simulink model "ModelResonant"  (R2020b)
settings: Solver=ode45  StartTime=0.0  StopTime=5  RelTol=1e-3
settings Model: Creator=umberto  LastModifiedBy=umberto

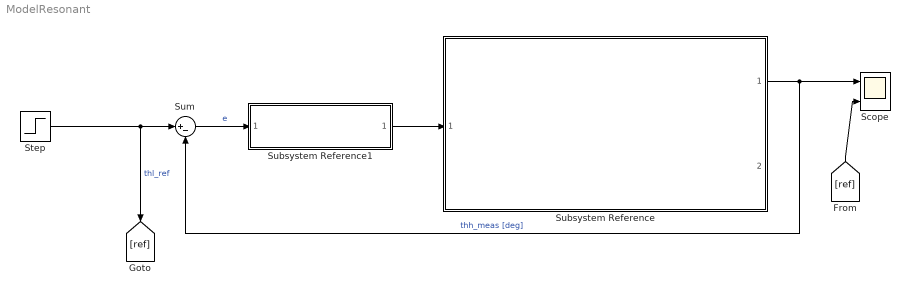
== system ModelResonant ==
  Scope : Scope  NumInputPorts=2
  Step : Step  Time=0  After=50  SampleTime=0
  Subsystem Reference : Subsystem  ReferencedSubsystem=DCServoMotor_SubSystem
  Subsystem Reference1 : Subsystem  ReferencedSubsystem=PID_SubSystem
  Sum : Sum  Inputs=|+-
  wires:
  Subsystem Reference/1 -> Sum/2, Scope/1  "thh_meas [deg]"
  Step/1 -> [ref], Sum/1  "thl_ref"
  Sum/1 -> Subsystem Reference1/1  "e"
  [ref] -> Scope/2
  Subsystem Reference1/1 -> Subsystem Reference/1
